simulink model "simulator"  (R2023b)
settings: configuration reference "SharedConfiguration" (kept outside this file)
undefined symbols (not defined in the file or in its folder): DiscIntNeverNeededParam
libraries: simulink x20
(part 1 of 2)
settings Model: DataDictionary=SharedDataDictionary.sldd  PacingRate=0.001000  VariantFading=off  Creator=hubkapatrik  LastModifiedBy=Ja
settings ConfigSetRef: SourceName=SharedConfiguration

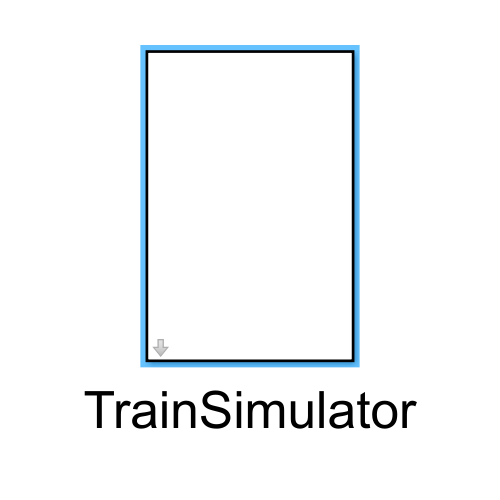
[thumbnail: Simulink's stored preview of the top-level diagram]
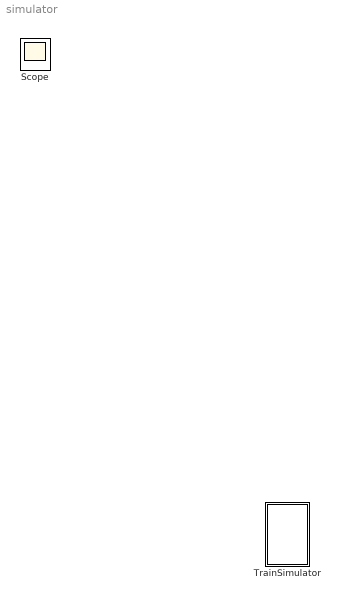
== system simulator ==
  TrainSimulator : Subsystem  mask{VelocityStart=10, MethodOfSpeedChange=constant acceleration, VelocityReq=10, Acceleration=1, PowerMaximum=3, PowerRelative=0.060, TractionForce=300, RoadResistEnable=yes, Gradient=0, CI_AfterReset=1, CI_Overreading=5.0, CI_Underreading=5.0, DrivingDirection=nominal}
      mask prompts: VelocityStart "Initial velocity"; MethodOfSpeedChange "Method of speed change"; VelocityReq "Required velocity"; PowerMaximum "Maximum power [MW]"; PowerRelative "Relative power [-]"; TractionForce "Traction force [kN]"; RoadResistEnable "Road resist enable"; Gradient "Gradient [‰]"; CI_AfterReset "Initial CI [%]"; CI_Overreading "CI overreading [%]"; CI_Underreading "CI underreading [%]"; DrivingDirection "Direction of train"
      mask TypeOptions MethodOfSpeedChange: constant velocity | sudden change of velocity | constant acceleration | break curves (not finished) | traction characteristics (not finished)
      mask TypeOptions RoadResistEnable: yes | no
      mask TypeOptions DrivingDirection: nominal | reverse
      mask DialogControl Container2 Prompt: Constant Acceleration
      mask DialogControl Container3 Prompt: Traction Characteristics
      mask DialogControl Container4 Prompt: Confidence Interval
  Scope : Scope

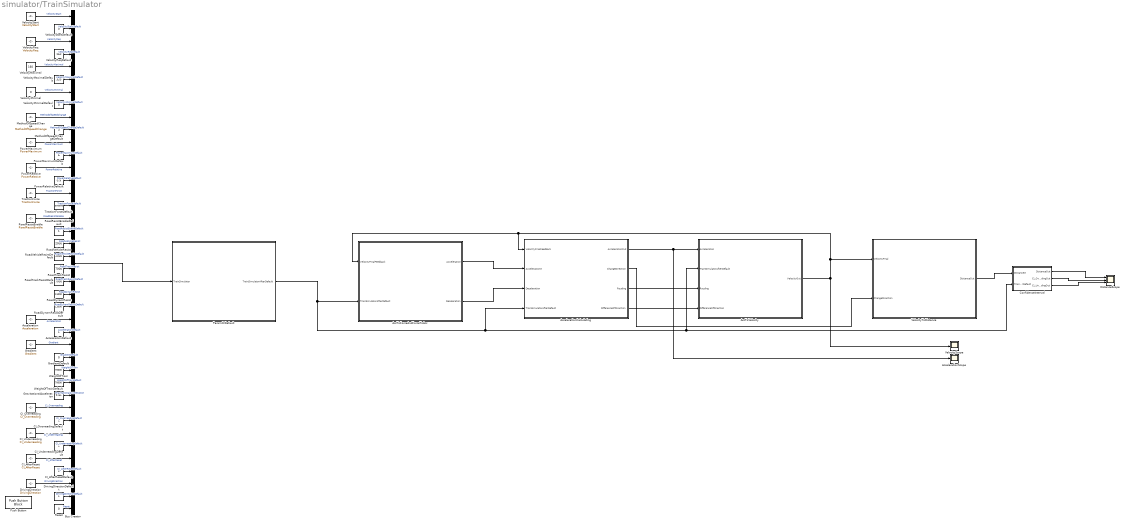
== system simulator/TrainSimulator ==
  AccToForceAndForceToAcc : Subsystem
  AccToVelocity : Subsystem
  Acceleration : Constant  Value=Acceleration  VectorParams1D=off  OutDataTypeStr=double
  AccelerationCalculating : Subsystem
  AccelerationDefault : Constant  VectorParams1D=off  OutDataTypeStr=double
  AccelerationScope : Scope
  Bus Creator : BusCreator  Inputs=VelocityStart,VelocityStartDefault,VelocityReq,VelocityReqDefault,VelocityMaximal,VelocityMaximalDefault,VelocityMinimal,VelocityMinimalDefault,MethodOfSpeedChange,MethodOfSpeedChangeDefault,PowerMaximum,PowerMaximumDefault,PowerRelative,PowerRelativeDefault,TractionForce,TractionForceDefault,RoadResistEnable,RoadResistEnableDefault,RoadVehicleResist,RoadVehicleResistDefault,RoadTrackResist,RoadTrackResistDefault,RoadDynamResist,RoadDynamResistDefault,Acceleration,AccelerationDefault,Gradient,GradientDefault,WeightOfTrain,WeightOfTrainDefault,GravitationalAcceleration,CI_Overreading,CI_OverreadingDefault,CI_Underreading,CI_UnderreadingDefault,CI_AfterReset,CI_AfterResetDefault,DrivingDirection,DrivingDirectionDefault,Reset  OutDataTypeStr=Bus: TrainSimulator  NonVirtualBus=on
  CI_AfterReset : Constant  Value=CI_AfterReset
  CI_AfterResetDefault : Constant  OutDataTypeStr=double
  CI_Overreading : Constant  Value=CI_Overreading
  CI_OverreadingDefault : Constant  OutDataTypeStr=double
  CI_Underreading : Constant  Value=CI_Underreading
  CI_UnderreadingDefault : Constant  OutDataTypeStr=double
  ConfidenceInterval : Subsystem
  DistanceScope : Scope  NumInputPorts=3
  DrivingDirection : Constant  Value=DrivingDirection  OutMin=0  OutMax=2  OutDataTypeStr=uint8
  DrivingDirectionDefault : Constant  OutMin=0  OutMax=2  OutDataTypeStr=uint8
  Gradient : Constant  Value=Gradient  OutDataTypeStr=double
  GradientDefault : Constant  Value=0  OutDataTypeStr=double
  GravitationalAcceleration : Constant  Value=9.81  OutMin=0  OutDataTypeStr=double
  MethodOfSpeedChange : Constant  Value=MethodOfSpeedChange  VectorParams1D=off  OutMin=1  OutMax=5  OutDataTypeStr=double
  MethodOfSpeedChangeDefault : Constant  Value=3  OutMin=1  OutMax=5  OutDataTypeStr=double
  ParamOrDefault : Subsystem
  PowerMaximum : Constant  Value=PowerMaximum
  PowerMaximumDefault : Constant  Value=6
  PowerRelative : Constant  Value=PowerRelative
  PowerRelativeDefault : Constant  Value=0.9
  Push Button : PushButtonBlock  OffValue=0.000000
  Reset : Constant  Value=0  OutMin=0  OutMax=1  OutDataTypeStr=double
  RoadDynamResist : Constant  Value=11000  OutMin=0  OutDataTypeStr=double
  RoadDynamResistDefault : Constant  Value=11000  VectorParams1D=off  OutMin=0  OutDataTypeStr=double
  RoadResistEnable : Constant  Value=RoadResistEnable  OutMin=0  OutMax=2  OutDataTypeStr=double
  RoadResistEnableDefault : Constant  OutMin=0  OutMax=1  OutDataTypeStr=double
  RoadTrackResist : Constant  Value=7000  OutMin=0  OutDataTypeStr=double
  RoadTrackResistDefault : Constant  Value=7000  OutMin=0  OutDataTypeStr=double
  RoadVehicleResist : Constant  Value=2000  OutMin=0  OutDataTypeStr=double
  RoadVehicleResistDefault : Constant  Value=2000  OutMin=0  OutDataTypeStr=double
  TractionForce : Constant  Value=TractionForce
  TractionForceDefault : Constant  Value=300000
  VelocityMaximal : Constant  Value=160  OutMin=0  OutDataTypeStr=double
  VelocityMaximalDefault : Constant  Value=320  OutMin=0  OutDataTypeStr=double
  VelocityMinimal : Constant  Value=0  OutMin=0  OutDataTypeStr=double
  VelocityMinimalDefault : Constant  Value=0  OutMin=0  OutDataTypeStr=double
  VelocityReq : Constant  Value=VelocityReq  OutMin=0  OutDataTypeStr=double
  VelocityReqDefault : Constant  Value=160  OutMin=0  OutDataTypeStr=double
  VelocityScope : Scope
  VelocityStart : Constant  Value=VelocityStart  OutMin=0  OutDataTypeStr=double
  VelocityStartDefault : Constant  Value=0  OutMin=0  OutDataTypeStr=double
  VelocityToDistance : Subsystem
  WeightOfTrain : Constant  Value=70000  OutMin=0  OutDataTypeStr=double
  WeightOfTrainDefault : Constant  Value=70000  OutMin=0  OutDataTypeStr=double
  wires:
  MethodOfSpeedChange/1 -> Bus Creator/9  "MethodOfSpeedChange"
  VelocityReq/1 -> Bus Creator/3  "VelocityReq"
  VelocityToDistance/1(DistanceOut) -> ConfidenceInterval/1(DistanceIn)
  Reset/1 -> Bus Creator/40  "Reset"
  VelocityStartDefault/1 -> Bus Creator/2  "VelocityStartDefault"
  Bus Creator/1 -> ParamOrDefault/1(TrainSimulator)
  DrivingDirectionDefault/1 -> Bus Creator/39  "DrivingDirectionDefault"
  RoadDynamResistDefault/1 -> Bus Creator/24  "RoadDynamResistDefault"
  RoadTrackResist/1 -> Bus Creator/21  "RoadTrackResist"
  RoadResistEnable/1 -> Bus Creator/17  "RoadResistEnable"
  RoadDynamResist/1 -> Bus Creator/23  "RoadDynamResist"
  RoadVehicleResist/1 -> Bus Creator/19  "RoadVehicleResist"
  Acceleration/1 -> Bus Creator/25  "Acceleration"
  ParamOrDefault/1(TrainSimulatorAfterDefault) -> ConfidenceInterval/2(TrainSimulatorAfterDefault), AccToVelocity/2(TrainSimulatorAfterDefault), AccelerationCalculating/4(TrainSimulatorAfterDefault), AccToForceAndForceToAcc/2(TrainSimulatorAfterDefault)
  WeightOfTrain/1 -> Bus Creator/29  "WeightOfTrain"
  RoadResistEnableDefault/1 -> Bus Creator/18  "RoadResistEnableDefault"
  GravitationalAcceleration/1 -> Bus Creator/31  "GravitationalAcceleration"
  MethodOfSpeedChangeDefault/1 -> Bus Creator/10  "MethodOfSpeedChangeDefault"
  GradientDefault/1 -> Bus Creator/28  "GradientDefault"
  AccelerationCalculating/1(AccelerationOut) -> AccelerationScope/1, AccToVelocity/1(Acceleration)
  RoadTrackResistDefault/1 -> Bus Creator/22  "RoadTrackResistDefault"
  VelocityReqDefault/1 -> Bus Creator/4  "VelocityReqDefault"
  WeightOfTrainDefault/1 -> Bus Creator/30  "WeightOfTrainDefault"
  AccToForceAndForceToAcc/1(Acceleration) -> AccelerationCalculating/2(AccelerationIn)
  Gradient/1 -> Bus Creator/27  "Gradient"
  AccelerationCalculating/2(ChangeDirection) -> VelocityToDistance/2(ChangeDirection)
  DrivingDirection/1 -> Bus Creator/38  "DrivingDirection"
  VelocityStart/1 -> Bus Creator/1  "VelocityStart"
  RoadVehicleResistDefault/1 -> Bus Creator/20  "RoadVehicleResistDefault"
  VelocityMinimal/1 -> Bus Creator/7  "VelocityMinimal"
  VelocityMinimalDefault/1 -> Bus Creator/8  "VelocityMinimalDefault"
  AccToForceAndForceToAcc/2(Deceleration) -> AccelerationCalculating/3(Deceleration)
  VelocityMaximal/1 -> Bus Creator/5  "VelocityMaximal"
  VelocityMaximalDefault/1 -> Bus Creator/6  "VelocityMaximalDefault"
  AccToVelocity/1(VelocityOut) -> AccelerationCalculating/1(VelocityFinalFeedback), AccToForceAndForceToAcc/1(VelocityFinalFeedback), VelocityToDistance/1(VelocityFinal), VelocityScope/1
  PowerRelative/1 -> Bus Creator/13  "PowerRelative"
  PowerRelativeDefault/1 -> Bus Creator/14  "PowerRelativeDefault"
  PowerMaximumDefault/1 -> Bus Creator/12  "PowerMaximumDefault"
  PowerMaximum/1 -> Bus Creator/11  "PowerMaximum"
  TractionForceDefault/1 -> Bus Creator/16  "TractionForceDefault"
  TractionForce/1 -> Bus Creator/15  "TractionForce"
  AccelerationCalculating/3(Rouding) -> AccToVelocity/3(Rouding)
  AccelerationCalculating/4(DifferenceOfDirection) -> AccToVelocity/4(DifferenceOfDirection)
  CI_Overreading/1 -> Bus Creator/32  "CI_Overreading"
  CI_Underreading/1 -> Bus Creator/34  "CI_Underreading"
  CI_AfterReset/1 -> Bus Creator/36  "CI_AfterReset"
  ConfidenceInterval/1(DistanceOut) -> DistanceScope/1
  ConfidenceInterval/2(CI_OverreadingOut) -> DistanceScope/2
  ConfidenceInterval/3(CI_UnderreadingOut) -> DistanceScope/3
  AccelerationDefault/1 -> Bus Creator/26  "AccelerationDefault"
  CI_OverreadingDefault/1 -> Bus Creator/33  "CI_OverreadingDefault"
  CI_UnderreadingDefault/1 -> Bus Creator/35  "CI_UnderreadingDefault"
  CI_AfterResetDefault/1 -> Bus Creator/37  "CI_AfterResetDefault"

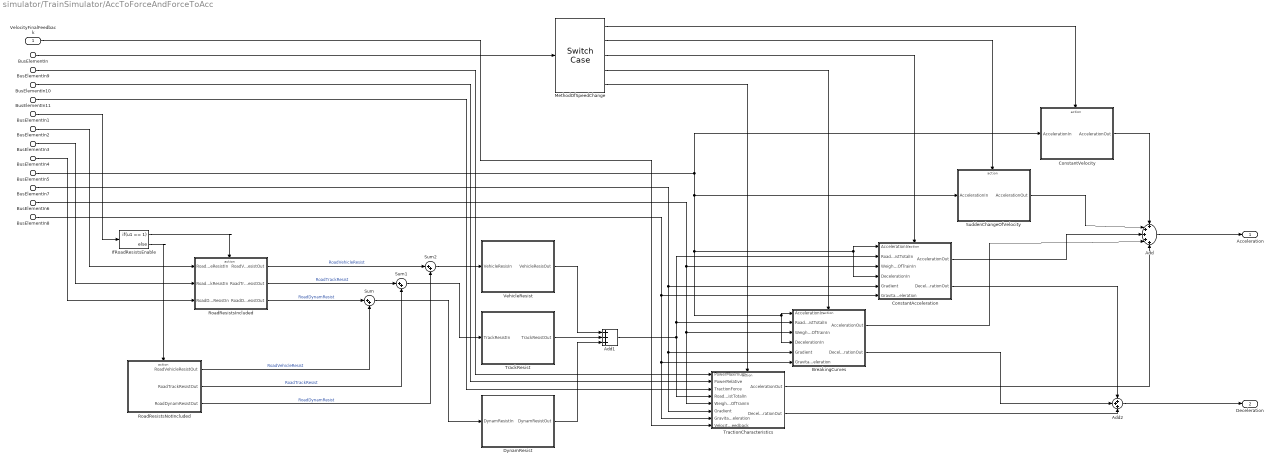
== system simulator/TrainSimulator/AccToForceAndForceToAcc ==
  VelocityFinalFeedback : Inport
  BusElementIn : Inport  Port=2  PortName=TrainSimulatorAfterDefault  Element=MethodOfSpeedChange
  BusElementIn9 : Inport  Port=2  PortName=TrainSimulatorAfterDefault  Element=PowerMaximum
  BusElementIn10 : Inport  Port=2  PortName=TrainSimulatorAfterDefault  Element=PowerRelative
  BusElementIn11 : Inport  Port=2  PortName=TrainSimulatorAfterDefault  Element=TractionForce
  BusElementIn1 : Inport  Port=2  PortName=TrainSimulatorAfterDefault  Element=RoadResistEnable
  BusElementIn2 : Inport  Port=2  PortName=TrainSimulatorAfterDefault  Element=RoadVehicleResist
  BusElementIn3 : Inport  Port=2  PortName=TrainSimulatorAfterDefault  Element=RoadTrackResist
  BusElementIn4 : Inport  Port=2  PortName=TrainSimulatorAfterDefault  Element=RoadDynamResist
  BusElementIn5 : Inport  Port=2  PortName=TrainSimulatorAfterDefault  Element=Acceleration
  BusElementIn7 : Inport  Port=2  PortName=TrainSimulatorAfterDefault  Element=Gradient
  BusElementIn6 : Inport  Port=2  PortName=TrainSimulatorAfterDefault  Element=WeightOfTrain
  BusElementIn8 : Inport  Port=2  PortName=TrainSimulatorAfterDefault  Element=GravitationalAcceleration
  Add : Sum  Inputs=+++++  OutDataTypeStr=double  AccumDataTypeStr=double
  Add1 : Sum  Inputs=+++  OutMin=0  OutDataTypeStr=double  AccumDataTypeStr=double
  Add2 : Sum  Inputs=+++  OutDataTypeStr=double  AccumDataTypeStr=double
  BreakingCurves : Subsystem
  ConstantAcceleration : Subsystem
  ConstantVelocity : Subsystem
  DynamResist : Subsystem
  IfRoadResistsEnable : If  IfExpression=u1 == 1
  MethodOfSpeedChange : SwitchCase  CaseConditions={1,2,3,4,5}  ShowDefaultCase=off
  RoadResistsIncluded : Subsystem
  RoadResistsNotIncluded : Subsystem
  SuddenChangeOfVelocity : Subsystem
  Sum : Sum  Inputs=|++  OutMin=0  AccumDataTypeStr=double
  Sum1 : Sum  Inputs=|++  OutMin=0  AccumDataTypeStr=double
  Sum2 : Sum  Inputs=|++  OutMin=0  AccumDataTypeStr=double
  TrackResist : Subsystem
  TractionCharacteristics : Subsystem
  VehicleResist : Subsystem
  Acceleration : Outport  OutDataTypeStr=double
  Deceleration : Outport  Port=2  OutDataTypeStr=double
  wires:
  BusElementIn/1 -> MethodOfSpeedChange/1
  MethodOfSpeedChange/5 -> TractionCharacteristics/Action
  MethodOfSpeedChange/4 -> BreakingCurves/Action
  MethodOfSpeedChange/3 -> ConstantAcceleration/Action
  MethodOfSpeedChange/2 -> SuddenChangeOfVelocity/Action
  MethodOfSpeedChange/1 -> ConstantVelocity/Action
  BusElementIn5/1 -> BreakingCurves/4(DecelerationIn), BreakingCurves/1(AccelerationIn), ConstantAcceleration/4(DecelerationIn), ConstantAcceleration/1(AccelerationIn), SuddenChangeOfVelocity/1(AccelerationIn), ConstantVelocity/1(AccelerationIn)
  ConstantVelocity/1(AccelerationOut) -> Add/1
  ConstantAcceleration/1(AccelerationOut) -> Add/3
  BreakingCurves/1(AccelerationOut) -> Add/4
  TractionCharacteristics/1(AccelerationOut) -> Add/5
  IfRoadResistsEnable/1 -> RoadResistsIncluded/Action
  IfRoadResistsEnable/2 -> RoadResistsNotIncluded/Action
  RoadResistsNotIncluded/1(RoadVehicleResistOut) -> Sum/2  "RoadVehicleResist"
  RoadResistsNotIncluded/2(RoadTrackResistOut) -> Sum1/2  "RoadTrackResist"
  RoadResistsNotIncluded/3(RoadDynamResistOut) -> Sum2/2  "RoadDynamResist"
  RoadResistsIncluded/1(RoadVehicleResistOut) -> Sum2/1  "RoadVehicleResist"
  RoadResistsIncluded/2(RoadTrackResistOut) -> Sum1/1  "RoadTrackResist"
  RoadResistsIncluded/3(RoadDynamResistOut) -> Sum/1  "RoadDynamResist"
  SuddenChangeOfVelocity/1(AccelerationOut) -> Add/2
  VehicleResist/1(VehicleResisOut) -> Add1/1
  TrackResist/1(TrackResistOut) -> Add1/2
  DynamResist/1(DynamResistOut) -> Add1/3
  Add1/1 -> BreakingCurves/2(RoadResistTotalIn), ConstantAcceleration/2(RoadResistTotalIn), TractionCharacteristics/4(RoadResistTotalIn)
  BusElementIn1/1 -> IfRoadResistsEnable/1
  BusElementIn2/1 -> RoadResistsIncluded/1(RoadVehicleResistIn)
  BusElementIn3/1 -> RoadResistsIncluded/2(RoadTrackResistIn)
  BusElementIn4/1 -> RoadResistsIncluded/3(RoadDynamResistIn)
  BusElementIn6/1 -> ConstantAcceleration/3(WeightOfTrainIn), BreakingCurves/3(WeightOfTrainIn), TractionCharacteristics/5(WeightOfTrainIn)
  ConstantAcceleration/2(DecelerationOut) -> Add2/1
  BreakingCurves/2(DecelerationOut) -> Add2/2
  TractionCharacteristics/2(DecelerationOut) -> Add2/3
  Sum/1 -> DynamResist/1(DynamResistIn)
  Sum1/1 -> TrackResist/1(TrackResistIn)
  Sum2/1 -> VehicleResist/1(VehicleResisIn)
  BusElementIn7/1 -> ConstantAcceleration/5(Gradient), BreakingCurves/5(Gradient), TractionCharacteristics/6(Gradient)
  BusElementIn8/1 -> ConstantAcceleration/6(GravitationalAcceleration), BreakingCurves/6(GravitationalAcceleration), TractionCharacteristics/7(GravitationalAcceleration)
  BusElementIn11/1 -> TractionCharacteristics/3(TractionForce)
  BusElementIn10/1 -> TractionCharacteristics/2(PowerRelative)
  BusElementIn9/1 -> TractionCharacteristics/1(PowerMaximum)
  VelocityFinalFeedback/1 -> TractionCharacteristics/8(VelocityFinalFeedback)
  Add/1 -> Acceleration/1
  Add2/1 -> Deceleration/1

== system simulator/TrainSimulator/AccToVelocity ==
  Acceleration : Inport  OutDataTypeStr=double
  BusElementIn : Inport  Port=2  PortName=TrainSimulatorAfterDefault  Element=VelocityStart
  BusElementIn1 : Inport  Port=2  PortName=TrainSimulatorAfterDefault  Element=VelocityReq
  BusElementIn3 : Inport  Port=2  PortName=TrainSimulatorAfterDefault  Element=VelocityMaximal
  BusElementIn2 : Inport  Port=2  PortName=TrainSimulatorAfterDefault  Element=VelocityMinimal
  Rouding : Inport  Port=3
  DifferenceOfDirection : Inport  Port=4  OutDataTypeStr=boolean
  AND : Logic  AllPortsSameDT=off  OutDataTypeStr=boolean
  Delay : Delay  DelayLength=1  InitialConditionSource=Input port  InitialCondition=20
      settings: InputPortMap=u0,p4
  DynamicChangeLimitMaxMinVelocity : Subsystem
  Switch : Switch  Criteria=u2 > Threshold  SaturateOnIntegerOverflow=off  InputSameDT=off
  VelocityOut : Outport  OutDataTypeStr=double
  wires:
  BusElementIn/1 -> Delay/2, DynamicChangeLimitMaxMinVelocity/3(VelocityStart)
  BusElementIn2/1 -> DynamicChangeLimitMaxMinVelocity/4(VelocityMinimal)
  Acceleration/1 -> DynamicChangeLimitMaxMinVelocity/1(Acceleration)
  BusElementIn3/1 -> DynamicChangeLimitMaxMinVelocity/2(VelocityMaxial)
  BusElementIn1/1 -> Switch/1
  Delay/1 -> VelocityOut/1
  DynamicChangeLimitMaxMinVelocity/1(VelocityOut) -> Switch/3
  AND/1 -> Switch/2
  DifferenceOfDirection/1 -> AND/1
  Switch/1 -> Delay/1
  Rouding/1 -> AND/2

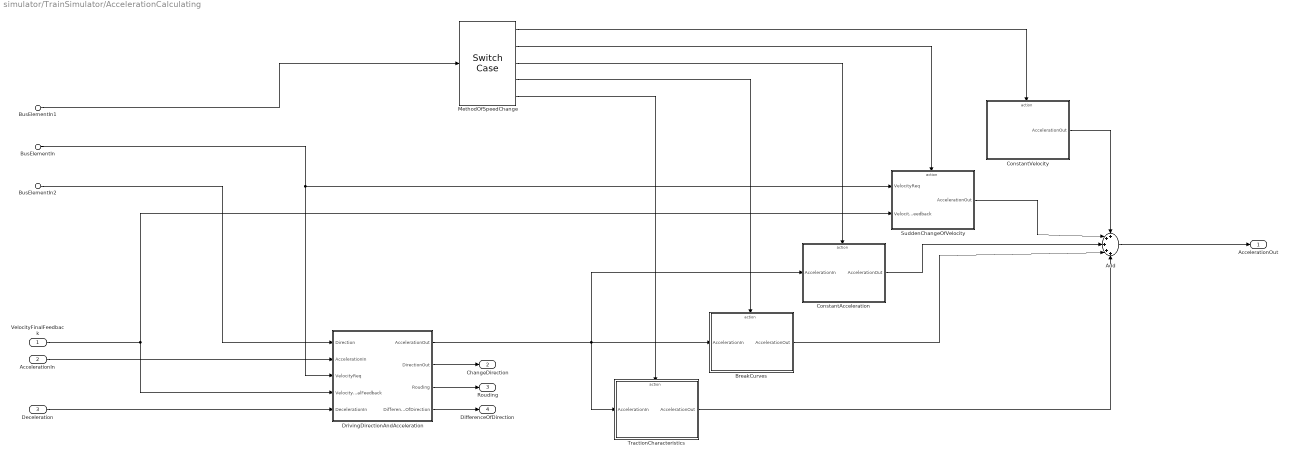
== system simulator/TrainSimulator/AccelerationCalculating ==
  VelocityFinalFeedback : Inport  OutDataTypeStr=double
  AccelerationIn : Inport  Port=2  OutDataTypeStr=double
  Deceleration : Inport  Port=3  OutDataTypeStr=double
  BusElementIn : Inport  Port=4  PortName=TrainSimulatorAfterDefault  Element=VelocityReq
  BusElementIn1 : Inport  Port=4  PortName=TrainSimulatorAfterDefault  Element=MethodOfSpeedChange
  BusElementIn2 : Inport  Port=4  PortName=TrainSimulatorAfterDefault  Element=DrivingDirection
  Add : Sum  Inputs=+++++  OutDataTypeStr=double  AccumDataTypeStr=double
  BreakCurves : Subsystem
  ConstantAcceleration : Subsystem
  ConstantVelocity : Subsystem
  DrivingDirectionAndAcceleration : Subsystem
  MethodOfSpeedChange : SwitchCase  CaseConditions={1,2,3,4,5}  ShowDefaultCase=off
  SuddenChangeOfVelocity : Subsystem
  TractionCharacteristics : Subsystem
  AccelerationOut : Outport  OutDataTypeStr=double
  ChangeDirection : Outport  Port=2  OutDataTypeStr=uint8
  Rouding : Outport  Port=3  OutDataTypeStr=double
  DifferenceOfDirection : Outport  Port=4  OutDataTypeStr=boolean
  wires:
  MethodOfSpeedChange/5 -> TractionCharacteristics/Action
  MethodOfSpeedChange/4 -> BreakCurves/Action
  MethodOfSpeedChange/3 -> ConstantAcceleration/Action
  MethodOfSpeedChange/1 -> ConstantVelocity/Action
  ConstantVelocity/1(AccelerationOut) -> Add/1
  SuddenChangeOfVelocity/1(AccelerationOut) -> Add/2
  ConstantAcceleration/1(AccelerationOut) -> Add/3
  TractionCharacteristics/1(AccelerationOut) -> Add/5
  MethodOfSpeedChange/2 -> SuddenChangeOfVelocity/Action
  BreakCurves/1(AccelerationOut) -> Add/4
  BusElementIn1/1 -> MethodOfSpeedChange/1
  BusElementIn2/1 -> DrivingDirectionAndAcceleration/1(Direction)
  BusElementIn/1 -> DrivingDirectionAndAcceleration/3(VelocityReq), SuddenChangeOfVelocity/1(VelocityReq)
  DrivingDirectionAndAcceleration/1(AccelerationOut) -> ConstantAcceleration/1(AccelerationIn), TractionCharacteristics/1(AccelerationIn), BreakCurves/1(AccelerationIn)
  AccelerationIn/1 -> DrivingDirectionAndAcceleration/2(AccelerationIn)
  VelocityFinalFeedback/1 -> DrivingDirectionAndAcceleration/4(VelocityFinalFeedback), SuddenChangeOfVelocity/2(VelocityFinalFeedback)
  Add/1 -> AccelerationOut/1
  DrivingDirectionAndAcceleration/2(DirectionOut) -> ChangeDirection/1
  Deceleration/1 -> DrivingDirectionAndAcceleration/5(DecelerationIn)
  DrivingDirectionAndAcceleration/3(Rouding) -> Rouding/1
  DrivingDirectionAndAcceleration/4(DifferenceOfDirection) -> DifferenceOfDirection/1

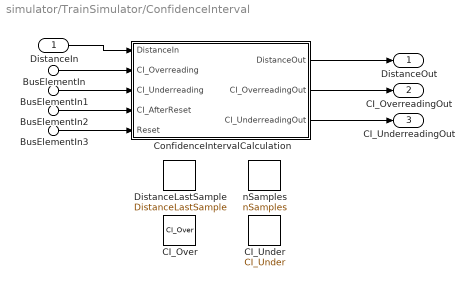
== system simulator/TrainSimulator/ConfidenceInterval ==
  DistanceIn : Inport  OutDataTypeStr=double
  BusElementIn : Inport  Port=2  PortName=TrainSimulatorAfterDefault  Element=CI_Overreading
  BusElementIn1 : Inport  Port=2  PortName=TrainSimulatorAfterDefault  Element=CI_Underreading
  BusElementIn2 : Inport  Port=2  PortName=TrainSimulatorAfterDefault  Element=CI_AfterReset
  BusElementIn3 : Inport  Port=2  PortName=TrainSimulatorAfterDefault  Element=Reset
  CI_Over : DataStoreMemory  DataStoreName=CI_Over  WriteAfterWriteMsg=warning  ShowAdditionalParam=off  OutDataTypeStr=double
  CI_Under : DataStoreMemory  DataStoreName=CI_Under  WriteAfterWriteMsg=warning  ShowAdditionalParam=off  OutDataTypeStr=double
  ConfidenceIntervalCalculation : MATLAB Function  TreatAsAtomicUnit=on
  DistanceLastSample : DataStoreMemory  DataStoreName=DistanceLastSample  WriteAfterWriteMsg=warning  ShowAdditionalParam=off  OutDataTypeStr=double
  nSamples : DataStoreMemory  DataStoreName=nSamples  WriteAfterWriteMsg=warning  ShowAdditionalParam=off  OutDataTypeStr=double
  DistanceOut : Outport
  CI_OverreadingOut : Outport  Port=2
  CI_UnderreadingOut : Outport  Port=3
  wires:
  BusElementIn3/1 -> ConfidenceIntervalCalculation/5(Reset)
  BusElementIn2/1 -> ConfidenceIntervalCalculation/4(CI_AfterReset)
  BusElementIn1/1 -> ConfidenceIntervalCalculation/3(CI_Underreading)
  BusElementIn/1 -> ConfidenceIntervalCalculation/2(CI_Overreading)
  DistanceIn/1 -> ConfidenceIntervalCalculation/1(DistanceIn)
  ConfidenceIntervalCalculation/2(CI_OverreadingOut) -> CI_OverreadingOut/1
  ConfidenceIntervalCalculation/1(DistanceOut) -> DistanceOut/1
  ConfidenceIntervalCalculation/3(CI_UnderreadingOut) -> CI_UnderreadingOut/1

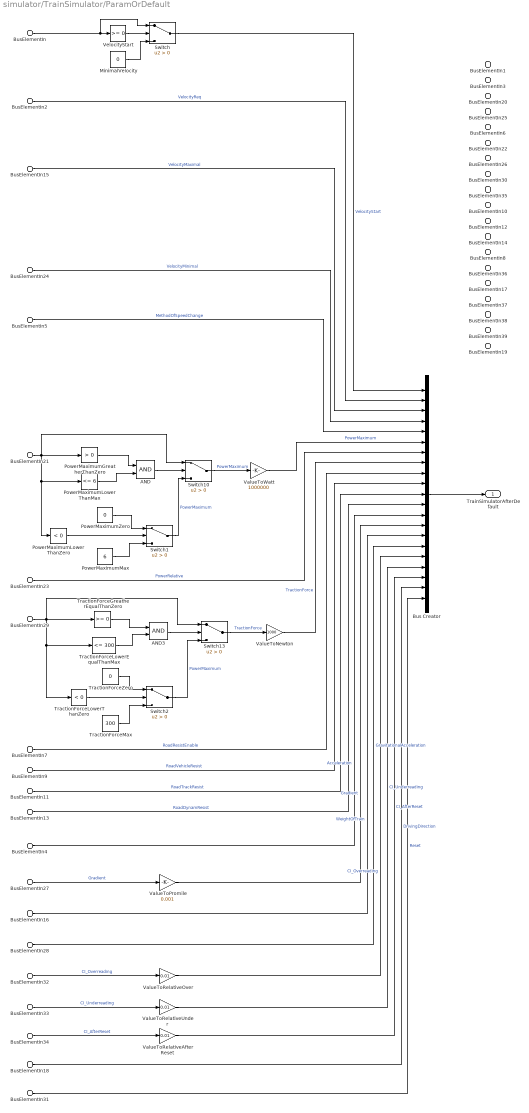
== system simulator/TrainSimulator/ParamOrDefault ==
  BusElementIn : Inport  PortName=TrainSimulator  Element=VelocityStart
  BusElementIn1 : Inport  PortName=TrainSimulator  Element=VelocityStartDefault
  BusElementIn2 : Inport  PortName=TrainSimulator  Element=VelocityReq
  BusElementIn3 : Inport  PortName=TrainSimulator  Element=VelocityReqDefault
  BusElementIn15 : Inport  PortName=TrainSimulator  Element=VelocityMaximal
  BusElementIn20 : Inport  PortName=TrainSimulator  Element=VelocityMaximalDefault
  BusElementIn24 : Inport  PortName=TrainSimulator  Element=VelocityMinimal
  BusElementIn25 : Inport  PortName=TrainSimulator  Element=VelocityMinimalDefault
  BusElementIn5 : Inport  PortName=TrainSimulator  Element=MethodOfSpeedChange
  BusElementIn6 : Inport  PortName=TrainSimulator  Element=MethodOfSpeedChangeDefault
  BusElementIn21 : Inport  PortName=TrainSimulator  Element=PowerMaximum
  BusElementIn22 : Inport  PortName=TrainSimulator  Element=PowerMaximumDefault
  BusElementIn23 : Inport  PortName=TrainSimulator  Element=PowerRelative
  BusElementIn26 : Inport  PortName=TrainSimulator  Element=PowerRelativeDefault
  BusElementIn29 : Inport  PortName=TrainSimulator  Element=TractionForce
  BusElementIn30 : Inport  PortName=TrainSimulator  Element=TractionForceDefault
  BusElementIn7 : Inport  PortName=TrainSimulator  Element=RoadResistEnable
  BusElementIn35 : Inport  PortName=TrainSimulator  Element=RoadResistEnableDefault
  BusElementIn9 : Inport  PortName=TrainSimulator  Element=RoadVehicleResist
  BusElementIn10 : Inport  PortName=TrainSimulator  Element=RoadVehicleResistDefault
  BusElementIn11 : Inport  PortName=TrainSimulator  Element=RoadTrackResist
  BusElementIn12 : Inport  PortName=TrainSimulator  Element=RoadTrackResistDefault
  BusElementIn13 : Inport  PortName=TrainSimulator  Element=RoadDynamResist
  BusElementIn14 : Inport  PortName=TrainSimulator  Element=RoadDynamResistDefault
  BusElementIn4 : Inport  PortName=TrainSimulator  Element=Acceleration
  BusElementIn8 : Inport  PortName=TrainSimulator  Element=AccelerationDefault
  BusElementIn27 : Inport  PortName=TrainSimulator  Element=Gradient
  BusElementIn36 : Inport  PortName=TrainSimulator  Element=GradientDefault
  BusElementIn16 : Inport  PortName=TrainSimulator  Element=WeightOfTrain
  BusElementIn17 : Inport  PortName=TrainSimulator  Element=WeightOfTrainDefault
  BusElementIn28 : Inport  PortName=TrainSimulator  Element=GravitationalAcceleration
  BusElementIn32 : Inport  PortName=TrainSimulator  Element=CI_Overreading
  BusElementIn37 : Inport  PortName=TrainSimulator  Element=CI_OverreadingDefault
  BusElementIn33 : Inport  PortName=TrainSimulator  Element=CI_Underreading
  BusElementIn38 : Inport  PortName=TrainSimulator  Element=CI_UnderreadingDefault
  BusElementIn34 : Inport  PortName=TrainSimulator  Element=CI_AfterReset
  BusElementIn39 : Inport  PortName=TrainSimulator  Element=CI_AfterResetDefault
  BusElementIn18 : Inport  PortName=TrainSimulator  Element=DrivingDirection
  BusElementIn19 : Inport  PortName=TrainSimulator  Element=DrivingDirectionDefault
  BusElementIn31 : Inport  PortName=TrainSimulator  Element=Reset
  AND : Logic  AllPortsSameDT=off  OutDataTypeStr=boolean
  AND3 : Logic  AllPortsSameDT=off  OutDataTypeStr=boolean
  Bus Creator : BusCreator  Inputs=21  OutDataTypeStr=Bus: TrainSimulatorAfterDefault  NonVirtualBus=on
  MinimalVelocity : Constant  Value=0  OutDataTypeStr=double
  PowerMaximumGreatherThanZero : simulink/Logic and Bit Operations/Compare To Constant  relop=>  const=0  OutDataTypeStr=boolean
  PowerMaximumLowerThanMax : simulink/Logic and Bit Operations/Compare To Constant  relop=<=  const=6  OutDataTypeStr=boolean
  PowerMaximumLowerThanZero : simulink/Logic and Bit Operations/Compare To Constant  relop=<  const=0  OutDataTypeStr=boolean
  PowerMaximumMax : Constant  Value=6  OutDataTypeStr=double
  PowerMaximumZero : Constant  Value=0  OutDataTypeStr=double
  Switch{,1..2,10} (4 alike) : Switch  Criteria=u2 > Threshold  OutMin=0  OutDataTypeStr=double  SaturateOnIntegerOverflow=off  InputSameDT=off
  Switch13 : Switch  Criteria=u2 > Threshold  OutMin=0  OutMax=1  OutDataTypeStr=double  SaturateOnIntegerOverflow=off  InputSameDT=off
  TractionForceGreatherEqualThanZero : simulink/Logic and Bit Operations/Compare To Constant  relop=>=  const=0  OutDataTypeStr=boolean
  TractionForceLowerEqualThanMax : simulink/Logic and Bit Operations/Compare To Constant  relop=<=  const=300  OutDataTypeStr=boolean
  TractionForceLowerThanZero : simulink/Logic and Bit Operations/Compare To Constant  relop=<  const=0  OutDataTypeStr=boolean
  TractionForceMax : Constant  Value=300  OutDataTypeStr=double
  TractionForceZero : Constant  Value=0  OutDataTypeStr=double
  ValueToNewton : Gain  Gain=1000  ParamDataTypeStr=double  OutDataTypeStr=double
  ValueToPromile : Gain  Gain=0.001  ParamDataTypeStr=double  OutDataTypeStr=double
  ValueToRelativeAfterReset : Gain  Gain=0.01  ParamDataTypeStr=double  OutDataTypeStr=double
  ValueToRelativeOver : Gain  Gain=0.01  ParamDataTypeStr=double  OutDataTypeStr=double
  ValueToRelativeUnder : Gain  Gain=0.01  ParamDataTypeStr=double  OutDataTypeStr=double
  ValueToWatt : Gain  Gain=1000000  ParamDataTypeStr=double  OutDataTypeStr=double
  VelocityStart : simulink/Logic and Bit Operations/Compare To Constant  relop=>=  const=0  OutDataTypeStr=boolean
  TrainSimulatorAfterDefault : Outport  OutDataTypeStr=Bus: TrainSimulatorAfterDefault
  wires:
  VelocityStart/1 -> Switch/2
  Switch/1 -> Bus Creator/1  "VelocityStart"
  BusElementIn2/1 -> Bus Creator/2  "VelocityReq"
  BusElementIn7/1 -> Bus Creator/9  "RoadResistEnable"
  BusElementIn9/1 -> Bus Creator/10  "RoadVehicleResist"
  BusElementIn11/1 -> Bus Creator/11  "RoadTrackResist"
  BusElementIn13/1 -> Bus Creator/12  "RoadDynamResist"
  BusElementIn4/1 -> Bus Creator/13  "Acceleration"
  BusElementIn16/1 -> Bus Creator/15  "WeightOfTrain"
  BusElementIn18/1 -> Bus Creator/20  "DrivingDirection"
  Bus Creator/1 -> TrainSimulatorAfterDefault/1
  BusElementIn5/1 -> Bus Creator/5  "MethodOfSpeedChange"
  BusElementIn/1 -> Switch/1, VelocityStart/1
  BusElementIn24/1 -> Bus Creator/4  "VelocityMinimal"
  BusElementIn15/1 -> Bus Creator/3  "VelocityMaximal"
  BusElementIn21/1 -> PowerMaximumGreatherThanZero/1, Switch10/1, PowerMaximumLowerThanZero/1, PowerMaximumLowerThanMax/1
  ValueToWatt/1 -> Bus Creator/6  "PowerMaximum"
  BusElementIn23/1 -> Bus Creator/7  "PowerRelative"
  BusElementIn28/1 -> Bus Creator/16  "GravitationalAcceleration"
  ValueToPromile/1 -> Bus Creator/14  "Gradient"
  TractionForceGreatherEqualThanZero/1 -> AND3/1
  TractionForceLowerEqualThanMax/1 -> AND3/2
  AND3/1 -> Switch13/2
  ValueToNewton/1 -> Bus Creator/8  "TractionForce"
  BusElementIn31/1 -> Bus Creator/21  "Reset"
  ValueToRelativeOver/1 -> Bus Creator/17  "CI_Overreading"
  ValueToRelativeUnder/1 -> Bus Creator/18  "CI_Underreading"
  ValueToRelativeAfterReset/1 -> Bus Creator/19  "CI_AfterReset"
  Switch10/1 -> ValueToWatt/1  "PowerMaximum"
  Switch13/1 -> ValueToNewton/1  "TractionForce"
  BusElementIn27/1 -> ValueToPromile/1  "Gradient"
  BusElementIn32/1 -> ValueToRelativeOver/1  "CI_Overreading"
  BusElementIn33/1 -> ValueToRelativeUnder/1  "CI_Underreading"
  BusElementIn34/1 -> ValueToRelativeAfterReset/1  "CI_AfterReset"
  MinimalVelocity/1 -> Switch/3
  PowerMaximumGreatherThanZero/1 -> AND/1
  PowerMaximumLowerThanMax/1 -> AND/2
  AND/1 -> Switch10/2
  PowerMaximumLowerThanZero/1 -> Switch1/2
  PowerMaximumZero/1 -> Switch1/1
  PowerMaximumMax/1 -> Switch1/3
  Switch1/1 -> Switch10/3  "PowerMaximum"
  Switch2/1 -> Switch13/3  "PowerMaximum"
  TractionForceZero/1 -> Switch2/1
  BusElementIn29/1 -> TractionForceGreatherEqualThanZero/1, Switch13/1, TractionForceLowerEqualThanMax/1, TractionForceLowerThanZero/1
  TractionForceMax/1 -> Switch2/3
  TractionForceLowerThanZero/1 -> Switch2/2

== system simulator/TrainSimulator/VelocityToDistance ==
  VelocityFinal : Inport  OutDataTypeStr=double
  ChangeDirection : Inport  Port=2  OutDataTypeStr=uint8
  AddOrSubtract : Switch  Criteria=u2 > Threshold  OutDataTypeStr=double  SaturateOnIntegerOverflow=off  InputSameDT=off
  DrivingDirectionNominal : simulink/Logic and Bit Operations/Compare To Constant  relop===  const=2  OutDataTypeStr=boolean
  IfReverseDirectionSubtract : Gain  Gain=-1  OutDataTypeStr=double
  VelocityToDistance : DiscreteIntegrator  IntegratorMethod=Integration: Trapezoidal  gainval=1  SampleTime=-1  OutDataTypeStr=double  ICPrevOutput=DiscIntNeverNeededParam  ICPrevScaledInput=DiscIntNeverNeededParam
  DistanceOut : Outport  OutDataTypeStr=double
  wires:
  VelocityToDistance/1 -> DistanceOut/1
  VelocityFinal/1 -> IfReverseDirectionSubtract/1, AddOrSubtract/3
  IfReverseDirectionSubtract/1 -> AddOrSubtract/1
  AddOrSubtract/1 -> VelocityToDistance/1
  ChangeDirection/1 -> DrivingDirectionNominal/1
  DrivingDirectionNominal/1 -> AddOrSubtract/2

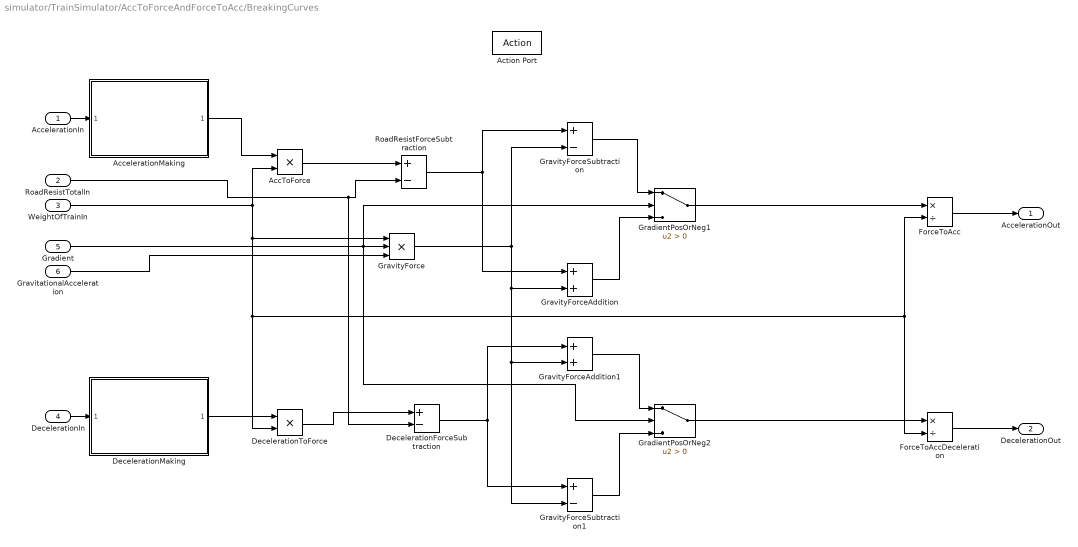
== system simulator/TrainSimulator/AccToForceAndForceToAcc/BreakingCurves ==
  AccelerationIn : Inport  OutDataTypeStr=double
  RoadResistTotalIn : Inport  Port=2  OutDataTypeStr=double
  WeightOfTrainIn : Inport  Port=3  OutDataTypeStr=double
  DecelerationIn : Inport  Port=4  OutDataTypeStr=double
  Gradient : Inport  Port=5
  GravitationalAcceleration : Inport  Port=6
  Action Port : ActionPort  ActionPortLabel=case [ 4 ]:
  AccToForce : Product  OutDataTypeStr=double
  AccelerationMaking : Subsystem  ReferencedSubsystem=AccelerationMaking
  DecelerationForceSubtraction : Sum  Inputs=+-  OutDataTypeStr=double  AccumDataTypeStr=double  RndMeth=Round
  DecelerationMaking : Subsystem  ReferencedSubsystem=DecelerationMaking
  DecelerationToForce : Product  OutDataTypeStr=double
  ForceToAcc : Product  Inputs=*/  OutDataTypeStr=double  RndMeth=Round
  ForceToAccDeceleration : Product  Inputs=*/  OutDataTypeStr=double  RndMeth=Round
  GradientPosOrNeg1 : Switch  Criteria=u2 > Threshold  OutDataTypeStr=double  SaturateOnIntegerOverflow=off  InputSameDT=off
  GradientPosOrNeg2 : Switch  Criteria=u2 > Threshold  OutDataTypeStr=double  SaturateOnIntegerOverflow=off  InputSameDT=off
  GravityForce : Product  Inputs=3  OutDataTypeStr=double
  GravityForceAddition : Sum  OutDataTypeStr=double  AccumDataTypeStr=double  RndMeth=Round
  GravityForceAddition1 : Sum  OutDataTypeStr=double  AccumDataTypeStr=double  RndMeth=Round
  GravityForceSubtraction : Sum  Inputs=+-  OutDataTypeStr=double  AccumDataTypeStr=double  RndMeth=Round
  GravityForceSubtraction1 : Sum  Inputs=+-  OutDataTypeStr=double  AccumDataTypeStr=double  RndMeth=Round
  RoadResistForceSubtraction : Sum  Inputs=+-  OutDataTypeStr=double  AccumDataTypeStr=double  RndMeth=Round
  AccelerationOut : Outport  OutDataTypeStr=double  OutputWhenDisabled=reset  InitialOutput=0
  DecelerationOut : Outport  Port=2  OutDataTypeStr=double  OutputWhenDisabled=reset  InitialOutput=0
  wires:
  DecelerationForceSubtraction/1 -> GravityForceAddition1/1, GravityForceSubtraction1/1
  GravityForceAddition1/1 -> GradientPosOrNeg2/1
  GravityForceSubtraction1/1 -> GradientPosOrNeg2/3
  GradientPosOrNeg2/1 -> ForceToAccDeceleration/1
  GravityForceAddition/1 -> GradientPosOrNeg1/3
  GradientPosOrNeg1/1 -> ForceToAcc/1
  GravityForceSubtraction/1 -> GradientPosOrNeg1/1
  GravityForce/1 -> GravityForceSubtraction/2, GravityForceAddition/2, GravityForceAddition1/2, GravityForceSubtraction1/2
  GravitationalAcceleration/1 -> GravityForce/3
  Gradient/1 -> GradientPosOrNeg1/2, GradientPosOrNeg2/2, GravityForce/2
  RoadResistForceSubtraction/1 -> GravityForceAddition/1, GravityForceSubtraction/1
  AccelerationMaking/1 -> AccToForce/1
  AccelerationIn/1 -> AccelerationMaking/1
  DecelerationMaking/1 -> DecelerationToForce/1
  DecelerationIn/1 -> DecelerationMaking/1
  ForceToAccDeceleration/1 -> DecelerationOut/1
  DecelerationToForce/1 -> DecelerationForceSubtraction/1
  RoadResistTotalIn/1 -> DecelerationForceSubtraction/2, RoadResistForceSubtraction/2
  ForceToAcc/1 -> AccelerationOut/1
  AccToForce/1 -> RoadResistForceSubtraction/1
  WeightOfTrainIn/1 -> AccToForce/2, ForceToAcc/2, ForceToAccDeceleration/2, DecelerationToForce/2, GravityForce/1

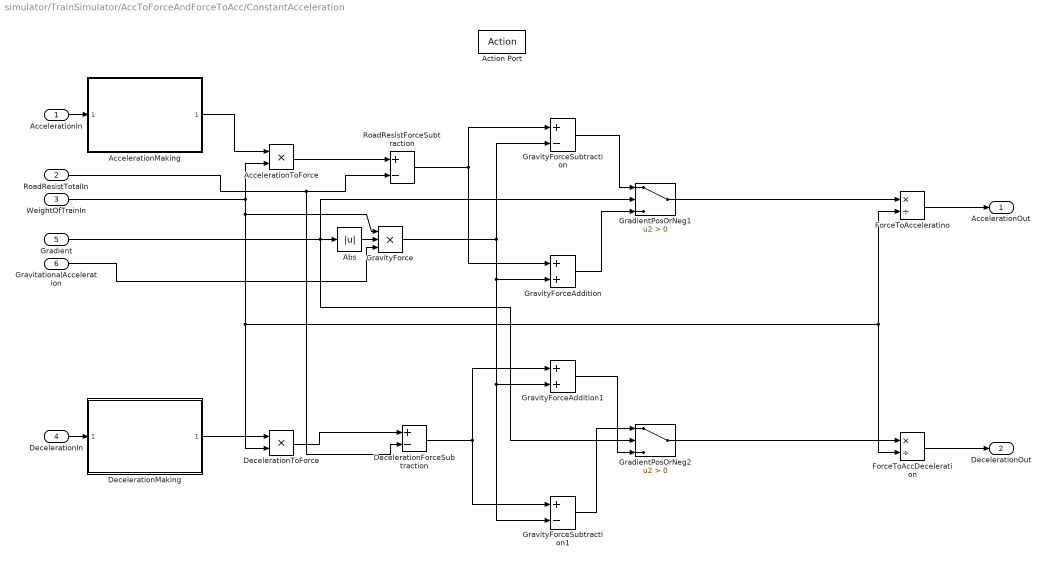
== system simulator/TrainSimulator/AccToForceAndForceToAcc/ConstantAcceleration ==
  AccelerationIn : Inport  OutDataTypeStr=double
  RoadResistTotalIn : Inport  Port=2  OutDataTypeStr=double
  WeightOfTrainIn : Inport  Port=3  OutDataTypeStr=double
  DecelerationIn : Inport  Port=4  OutDataTypeStr=double
  Gradient : Inport  Port=5
  GravitationalAcceleration : Inport  Port=6
  Action Port : ActionPort  ActionPortLabel=case [ 3 ]:
  Abs : Abs  OutDataTypeStr=double  SaturateOnIntegerOverflow=off
  AccelerationMaking : Subsystem  ReferencedSubsystem=AccelerationMaking
  AccelerationToForce : Product  OutDataTypeStr=double
  DecelerationForceSubtraction : Sum  Inputs=+-  OutDataTypeStr=double  AccumDataTypeStr=double  RndMeth=Round
  DecelerationMaking : Subsystem  ReferencedSubsystem=DecelerationMaking
  DecelerationToForce : Product  OutDataTypeStr=double
  ForceToAccDeceleration : Product  Inputs=*/  OutDataTypeStr=double  RndMeth=Round
  ForceToAcceleratino : Product  Inputs=*/  OutDataTypeStr=double  RndMeth=Round
  GradientPosOrNeg1 : Switch  Criteria=u2 > Threshold  OutDataTypeStr=double  SaturateOnIntegerOverflow=off  InputSameDT=off
  GradientPosOrNeg2 : Switch  Criteria=u2 > Threshold  OutDataTypeStr=double  SaturateOnIntegerOverflow=off  InputSameDT=off
  GravityForce : Product  Inputs=3  OutDataTypeStr=double
  GravityForceAddition : Sum  OutDataTypeStr=double  AccumDataTypeStr=double  RndMeth=Round
  GravityForceAddition1 : Sum  OutDataTypeStr=double  AccumDataTypeStr=double  RndMeth=Round
  GravityForceSubtraction : Sum  Inputs=+-  OutDataTypeStr=double  AccumDataTypeStr=double  RndMeth=Round
  GravityForceSubtraction1 : Sum  Inputs=+-  OutDataTypeStr=double  AccumDataTypeStr=double  RndMeth=Round
  RoadResistForceSubtraction : Sum  Inputs=+-  OutDataTypeStr=double  AccumDataTypeStr=double  RndMeth=Round
  AccelerationOut : Outport  OutDataTypeStr=double  OutputWhenDisabled=reset  InitialOutput=0
  DecelerationOut : Outport  Port=2  OutDataTypeStr=double  OutputWhenDisabled=reset  InitialOutput=0
  wires:
  WeightOfTrainIn/1 -> DecelerationToForce/2, ForceToAccDeceleration/2, ForceToAcceleratino/2, GravityForce/1, AccelerationToForce/2
  AccelerationToForce/1 -> RoadResistForceSubtraction/1
  ForceToAcceleratino/1 -> AccelerationOut/1
  RoadResistTotalIn/1 -> RoadResistForceSubtraction/2, DecelerationForceSubtraction/2
  DecelerationToForce/1 -> DecelerationForceSubtraction/1
  ForceToAccDeceleration/1 -> DecelerationOut/1
  DecelerationIn/1 -> DecelerationMaking/1
  DecelerationMaking/1 -> DecelerationToForce/1
  AccelerationIn/1 -> AccelerationMaking/1
  AccelerationMaking/1 -> AccelerationToForce/1
  RoadResistForceSubtraction/1 -> GravityForceSubtraction/1, GravityForceAddition/1
  GravitationalAcceleration/1 -> GravityForce/3
  GravityForce/1 -> GravityForceSubtraction1/2, GravityForceAddition1/2, GravityForceAddition/2, GravityForceSubtraction/2
  GravityForceSubtraction/1 -> GradientPosOrNeg1/1
  GradientPosOrNeg1/1 -> ForceToAcceleratino/1
  GravityForceAddition/1 -> GradientPosOrNeg1/3
  GradientPosOrNeg2/1 -> ForceToAccDeceleration/1
  GravityForceSubtraction1/1 -> GradientPosOrNeg2/1
  GravityForceAddition1/1 -> GradientPosOrNeg2/3
  DecelerationForceSubtraction/1 -> GravityForceSubtraction1/1, GravityForceAddition1/1
  Gradient/1 -> Abs/1, GradientPosOrNeg2/2, GradientPosOrNeg1/2
  Abs/1 -> GravityForce/2

== system simulator/TrainSimulator/AccToForceAndForceToAcc/ConstantVelocity ==
  AccelerationIn : Inport  OutDataTypeStr=double
  Action Port : ActionPort  ActionPortLabel=case [ 1 ]:
  AccelerationOut : Outport  OutDataTypeStr=double  OutputWhenDisabled=reset  InitialOutput=0
  wires:
  AccelerationIn/1 -> AccelerationOut/1

== system simulator/TrainSimulator/AccToForceAndForceToAcc/DynamResist ==
  DynamResistIn : Inport  OutMin=0  OutDataTypeStr=double
  DynamResistOut : Outport  OutMin=0  OutDataTypeStr=double
  wires:
  DynamResistIn/1 -> DynamResistOut/1

== system simulator/TrainSimulator/AccToForceAndForceToAcc/RoadResistsIncluded ==
  RoadVehicleResistIn : Inport  OutMin=0  OutDataTypeStr=double
  RoadTrackResistIn : Inport  Port=2  OutMin=0  OutDataTypeStr=double
  RoadDynamResistIn : Inport  Port=3  OutMin=0  OutDataTypeStr=double
  Action Port : ActionPort  ActionPortLabel=if(u1 == 1)
  RoadVehicleResistOut : Outport  OutMin=0  OutDataTypeStr=double  OutputWhenDisabled=reset  InitialOutput=0
  RoadTrackResistOut : Outport  Port=2  OutMin=0  OutDataTypeStr=double  OutputWhenDisabled=reset  InitialOutput=0
  RoadDynamResistOut : Outport  Port=3  OutMin=0  OutDataTypeStr=double  OutputWhenDisabled=reset  InitialOutput=0
  wires:
  RoadVehicleResistIn/1 -> RoadVehicleResistOut/1
  RoadTrackResistIn/1 -> RoadTrackResistOut/1
  RoadDynamResistIn/1 -> RoadDynamResistOut/1

== system simulator/TrainSimulator/AccToForceAndForceToAcc/RoadResistsNotIncluded ==
  Action Port : ActionPort  ActionPortLabel=else
  RoadDynamResistZero : Constant  Value=0  OutMin=0  OutMax=0  OutDataTypeStr=uint8
  RoadTrackResistZero : Constant  Value=0  OutMin=0  OutMax=0  OutDataTypeStr=uint8
  RoadVehicleResistZero : Constant  Value=0  OutMin=0  OutMax=0  OutDataTypeStr=uint8
  RoadVehicleResistOut : Outport  OutMin=0  OutMax=0  OutDataTypeStr=uint8  OutputWhenDisabled=reset  InitialOutput=0
  RoadTrackResistOut : Outport  Port=2  OutMin=0  OutMax=0  OutDataTypeStr=uint8  OutputWhenDisabled=reset  InitialOutput=0
  RoadDynamResistOut : Outport  Port=3  OutMin=0  OutMax=0  OutDataTypeStr=uint8  OutputWhenDisabled=reset  InitialOutput=0
  wires:
  RoadDynamResistZero/1 -> RoadDynamResistOut/1
  RoadVehicleResistZero/1 -> RoadVehicleResistOut/1
  RoadTrackResistZero/1 -> RoadTrackResistOut/1

== system simulator/TrainSimulator/AccToForceAndForceToAcc/SuddenChangeOfVelocity ==
  AccelerationIn : Inport  OutDataTypeStr=double
  Action Port : ActionPort  ActionPortLabel=case [ 2 ]:
  AccelerationOut : Outport  OutDataTypeStr=double  OutputWhenDisabled=reset  InitialOutput=0
  wires:
  AccelerationIn/1 -> AccelerationOut/1

== system simulator/TrainSimulator/AccToForceAndForceToAcc/TrackResist ==
  TrackResistIn : Inport  OutMin=0  OutDataTypeStr=double
  TrackResistOut : Outport  OutMin=0  OutDataTypeStr=double
  wires:
  TrackResistIn/1 -> TrackResistOut/1

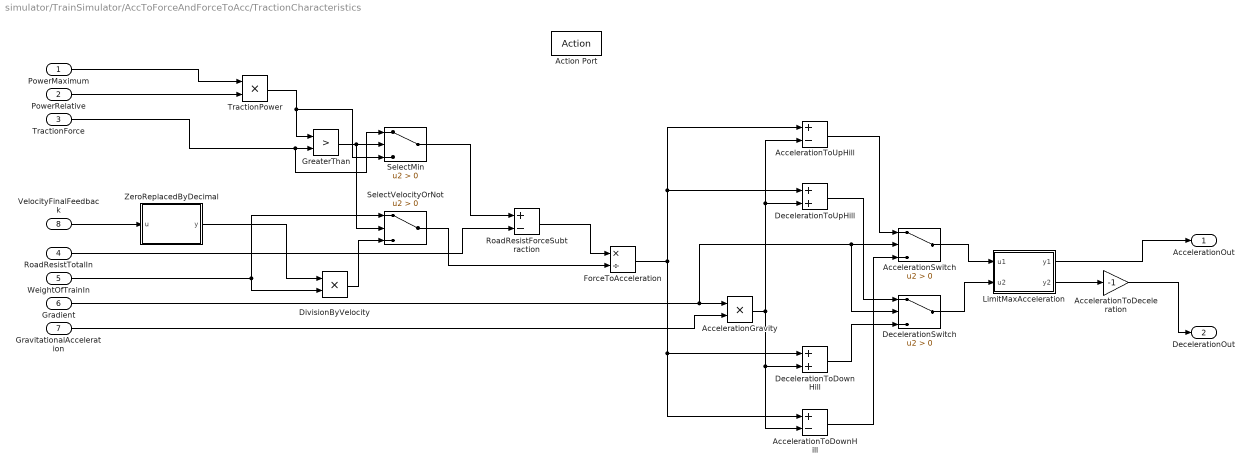
== system simulator/TrainSimulator/AccToForceAndForceToAcc/TractionCharacteristics ==
  PowerMaximum : Inport  OutDataTypeStr=double
  PowerRelative : Inport  Port=2  OutDataTypeStr=double
  TractionForce : Inport  Port=3  OutDataTypeStr=double
  RoadResistTotalIn : Inport  Port=4  OutDataTypeStr=double
  WeightOfTrainIn : Inport  Port=5  OutDataTypeStr=double
  Gradient : Inport  Port=6
  GravitationalAcceleration : Inport  Port=7
  VelocityFinalFeedback : Inport  Port=8
  Action Port : ActionPort  ActionPortLabel=case [ 5 ]:
  AccelerationGravity : Product  OutDataTypeStr=double
  AccelerationSwitch : Switch  Criteria=u2 > Threshold  SaturateOnIntegerOverflow=off  InputSameDT=off
  AccelerationToDeceleration : Gain  Gain=-1  ParamDataTypeStr=double
  AccelerationToDownHill : Sum  Inputs=+-
  AccelerationToUpHill : Sum  Inputs=+-
  DecelerationSwitch : Switch  Criteria=u2 > Threshold  SaturateOnIntegerOverflow=off  InputSameDT=off
  DecelerationToDownHill : Sum
  DecelerationToUpHill : Sum
  DivisionByVelocity : Product
  ForceToAcceleration : Product  Inputs=*/  OutDataTypeStr=double
  GreaterThan : RelationalOperator  Operator=>  OutDataTypeStr=boolean  RndMeth=Simplest  InputSameDT=off
  LimitMaxAcceleration : MATLAB Function  TreatAsAtomicUnit=on
  RoadResistForceSubtraction : Sum  Inputs=+-
  SelectMin : Switch  Criteria=u2 > Threshold  OutDataTypeStr=double  SaturateOnIntegerOverflow=off  InputSameDT=off
  SelectVelocityOrNot : Switch  Criteria=u2 > Threshold  OutDataTypeStr=double  SaturateOnIntegerOverflow=off  InputSameDT=off
  TractionPower : Product  OutDataTypeStr=double
  ZeroReplacedByDecimal : MATLAB Function  TreatAsAtomicUnit=on
  AccelerationOut : Outport  OutDataTypeStr=double  OutputWhenDisabled=reset  InitialOutput=0
  DecelerationOut : Outport  Port=2  OutDataTypeStr=double  OutputWhenDisabled=reset  InitialOutput=0
  wires:
  PowerRelative/1 -> TractionPower/2
  PowerMaximum/1 -> TractionPower/1
  TractionPower/1 -> SelectMin/3, GreaterThan/1
  TractionForce/1 -> SelectMin/1, GreaterThan/2
  SelectMin/1 -> RoadResistForceSubtraction/1
  Gradient/1 -> AccelerationSwitch/2, DecelerationSwitch/2, AccelerationGravity/1
  GravitationalAcceleration/1 -> AccelerationGravity/2
  ForceToAcceleration/1 -> DecelerationToDownHill/1, AccelerationToDownHill/1, DecelerationToUpHill/1, AccelerationToUpHill/1
  AccelerationGravity/1 -> DecelerationToUpHill/2, AccelerationToUpHill/2, DecelerationToDownHill/2, AccelerationToDownHill/2
  RoadResistForceSubtraction/1 -> ForceToAcceleration/1
  DecelerationToUpHill/1 -> DecelerationSwitch/1
  AccelerationToUpHill/1 -> AccelerationSwitch/1
  AccelerationToDeceleration/1 -> DecelerationOut/1
  AccelerationToDownHill/1 -> AccelerationSwitch/3
  DecelerationToDownHill/1 -> DecelerationSwitch/3
  RoadResistTotalIn/1 -> RoadResistForceSubtraction/2
  VelocityFinalFeedback/1 -> ZeroReplacedByDecimal/1(u)
  ZeroReplacedByDecimal/1(y) -> DivisionByVelocity/1
  GreaterThan/1 -> SelectVelocityOrNot/2, SelectMin/2
  DivisionByVelocity/1 -> SelectVelocityOrNot/3
  WeightOfTrainIn/1 -> SelectVelocityOrNot/1, DivisionByVelocity/2
  SelectVelocityOrNot/1 -> ForceToAcceleration/2
  DecelerationSwitch/1 -> LimitMaxAcceleration/2(u2)
  LimitMaxAcceleration/2(y2) -> AccelerationToDeceleration/1
  LimitMaxAcceleration/1(y1) -> AccelerationOut/1
  AccelerationSwitch/1 -> LimitMaxAcceleration/1(u1)

== system simulator/TrainSimulator/AccToForceAndForceToAcc/VehicleResist ==
  VehicleResisIn : Inport  OutMin=0  OutDataTypeStr=double
  VehicleResisOut : Outport  OutMin=0  OutDataTypeStr=double
  wires:
  VehicleResisIn/1 -> VehicleResisOut/1

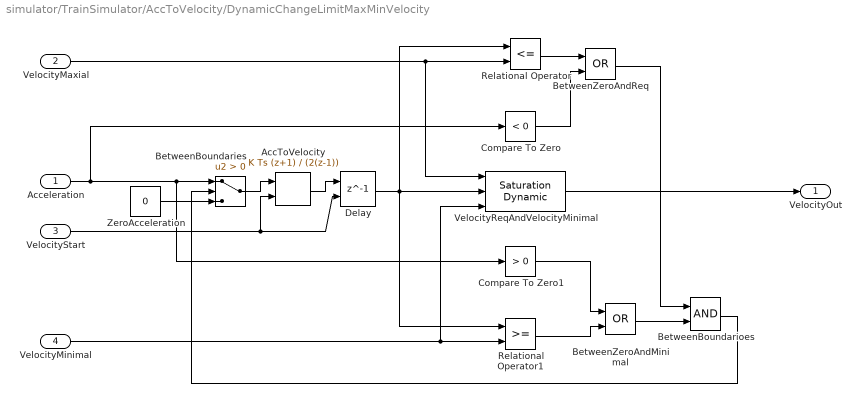
== system simulator/TrainSimulator/AccToVelocity/DynamicChangeLimitMaxMinVelocity ==
  Acceleration : Inport  OutDataTypeStr=double
  VelocityMaxial : Inport  Port=2  OutDataTypeStr=double
  VelocityStart : Inport  Port=3  OutDataTypeStr=double
  VelocityMinimal : Inport  Port=4  OutDataTypeStr=double
  AccToVelocity : DiscreteIntegrator  IntegratorMethod=Integration: Trapezoidal  InitialConditionSource=external  SampleTime=-1  OutDataTypeStr=double  UpperSaturationLimit=50  LowerSaturationLimit=0  ICPrevOutput=DiscIntNeverNeededParam  ICPrevScaledInput=DiscIntNeverNeededParam
  BetweenBoundaries : Switch  Criteria=u2 > Threshold  OutDataTypeStr=double  SaturateOnIntegerOverflow=off  InputSameDT=off
  BetweenBoundarioes : Logic  AllPortsSameDT=off  OutDataTypeStr=boolean
  BetweenZeroAndMinimal : Logic  Operator=OR  AllPortsSameDT=off  OutDataTypeStr=boolean
  BetweenZeroAndReq : Logic  Operator=OR  AllPortsSameDT=off  OutDataTypeStr=boolean
  Compare To Zero : simulink/Logic and Bit Operations/Compare To Zero  relop=<  OutDataTypeStr=boolean  ZeroCross=off
  Compare To Zero1 : simulink/Logic and Bit Operations/Compare To Zero  relop=>  OutDataTypeStr=boolean  ZeroCross=off
  Delay : Delay  DelayLength=1  InitialConditionSource=Input port
      settings: InputPortMap=u0,p4
  Relational Operator : RelationalOperator  Operator=<=  OutDataTypeStr=boolean  InputSameDT=off
  Relational Operator1 : RelationalOperator  OutDataTypeStr=boolean  InputSameDT=off
  VelocityReqAndVelocityMinimal : simulink/Discontinuities/Saturation Dynamic  OutMin=[]  OutMax=[]  OutDataTypeStr=double  OutDataType=fixdt(1, 16)  OutScaling=2^-10  RndMeth=Nearest  DoSatur=off
  ZeroAcceleration : Constant  Value=0  OutDataTypeStr=uint8
  VelocityOut : Outport  OutDataTypeStr=double
  wires:
  Acceleration/1 -> Compare To Zero1/1, BetweenBoundaries/1, Compare To Zero/1
  ZeroAcceleration/1 -> BetweenBoundaries/3
  BetweenBoundaries/1 -> AccToVelocity/1
  Relational Operator/1 -> BetweenZeroAndReq/1
  Compare To Zero/1 -> BetweenZeroAndReq/2
  VelocityMaxial/1 -> Relational Operator/2, VelocityReqAndVelocityMinimal/1
  VelocityMinimal/1 -> Relational Operator1/2, VelocityReqAndVelocityMinimal/3
  Compare To Zero1/1 -> BetweenZeroAndMinimal/1
  Relational Operator1/1 -> BetweenZeroAndMinimal/2
  BetweenZeroAndMinimal/1 -> BetweenBoundarioes/2
  BetweenZeroAndReq/1 -> BetweenBoundarioes/1
  BetweenBoundarioes/1 -> BetweenBoundaries/2
  VelocityReqAndVelocityMinimal/1 -> VelocityOut/1
  Delay/1 -> Relational Operator1/1, Relational Operator/1, VelocityReqAndVelocityMinimal/2
  VelocityStart/1 -> Delay/2, AccToVelocity/2
  AccToVelocity/1 -> Delay/1

== system simulator/TrainSimulator/AccelerationCalculating/BreakCurves ==
  AccelerationIn : Inport  OutDataTypeStr=double
  Action Port : ActionPort  ActionPortLabel=case [ 4 ]:
  AccelerationOut : Outport  OutDataTypeStr=double  InitialOutput=0
  wires:
  AccelerationIn/1 -> AccelerationOut/1

== system simulator/TrainSimulator/AccelerationCalculating/ConstantAcceleration ==
  AccelerationIn : Inport  OutDataTypeStr=double
  Action Port : ActionPort  ActionPortLabel=case [ 3 ]:
  AccelerationOut : Outport  OutDataTypeStr=double  InitialOutput=0
  wires:
  AccelerationIn/1 -> AccelerationOut/1

== system simulator/TrainSimulator/AccelerationCalculating/ConstantVelocity ==
  Action Port : ActionPort  ActionPortLabel=case [ 1 ]:
  ZeroAcceleration : Constant  Value=0  OutMin=0  OutMax=0  OutDataTypeStr=double
  AccelerationOut : Outport  OutDataTypeStr=double  InitialOutput=0
  wires:
  ZeroAcceleration/1 -> AccelerationOut/1

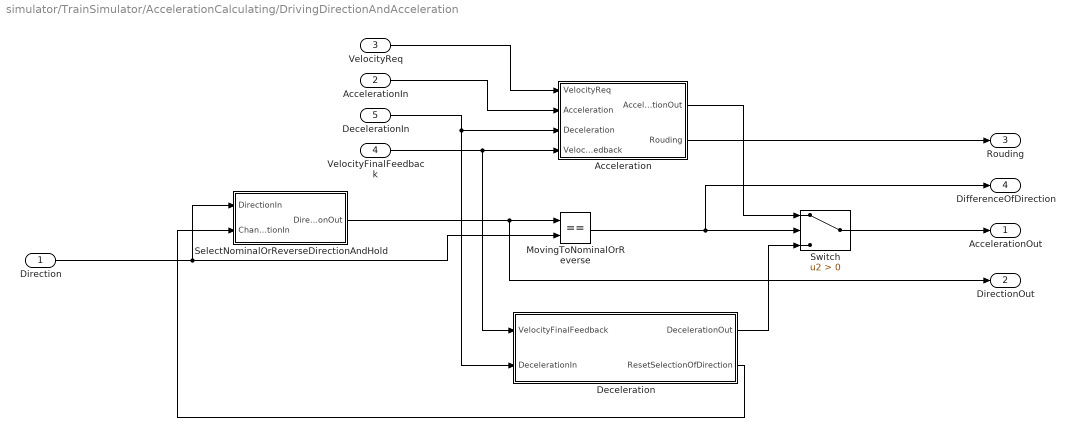
== system simulator/TrainSimulator/AccelerationCalculating/DrivingDirectionAndAcceleration ==
  Direction : Inport  OutDataTypeStr=uint8
  AccelerationIn : Inport  Port=2  OutDataTypeStr=double
  VelocityReq : Inport  Port=3  OutDataTypeStr=double
  VelocityFinalFeedback : Inport  Port=4  OutDataTypeStr=double
  DecelerationIn : Inport  Port=5  OutDataTypeStr=double
  Acceleration : Subsystem
  Deceleration : Subsystem
  MovingToNominalOrReverse : RelationalOperator  Operator===  OutDataTypeStr=boolean  RndMeth=Simplest  InputSameDT=off
  SelectNominalOrReverseDirectionAndHold : Subsystem
  Switch : Switch  Criteria=u2 > Threshold  OutDataTypeStr=double  SaturateOnIntegerOverflow=off  InputSameDT=off
  AccelerationOut : Outport  OutDataTypeStr=double  OutputWhenDisabled=reset  InitialOutput=0
  DirectionOut : Outport  Port=2  OutDataTypeStr=uint8  OutputWhenDisabled=reset  InitialOutput=0
  Rouding : Outport  Port=3  OutDataTypeStr=double
  DifferenceOfDirection : Outport  Port=4  OutDataTypeStr=boolean
  wires:
  Direction/1 -> MovingToNominalOrReverse/2, SelectNominalOrReverseDirectionAndHold/1(DirectionIn)
  SelectNominalOrReverseDirectionAndHold/1(DirectionOut) -> DirectionOut/1, MovingToNominalOrReverse/1
  MovingToNominalOrReverse/1 -> DifferenceOfDirection/1, Switch/2
  Deceleration/1(DecelerationOut) -> Switch/3
  Acceleration/1(AccelerationOut) -> Switch/1
  Switch/1 -> AccelerationOut/1
  VelocityFinalFeedback/1 -> Deceleration/1(VelocityFinalFeedback), Acceleration/4(VelocityFinalFeedback)
  VelocityReq/1 -> Acceleration/1(VelocityReq)
  Deceleration/2(ResetSelectionOfDirection) -> SelectNominalOrReverseDirectionAndHold/2(ChangeDirectionIn)
  DecelerationIn/1 -> Acceleration/3(Deceleration), Deceleration/2(DecelerationIn)
  AccelerationIn/1 -> Acceleration/2(Acceleration)
  Acceleration/2(Rouding) -> Rouding/1

== system simulator/TrainSimulator/AccelerationCalculating/SuddenChangeOfVelocity ==
  VelocityReq : Inport  OutDataTypeStr=double
  VelocityFinalFeedback : Inport  Port=2  OutDataTypeStr=double
  Action Port : ActionPort  ActionPortLabel=case [ 2 ]:
  Relational Operator1 : RelationalOperator  Operator=>  OutDataTypeStr=boolean  RndMeth=Simplest  InputSameDT=off
  Relational Operator2 : RelationalOperator  Operator=<  OutDataTypeStr=boolean  RndMeth=Simplest  InputSameDT=off
  SuddenChangeofSpeedToMax : Constant  Value=100000  OutDataTypeStr=uint32
  SuddenChangeofSpeedToMin : Constant  Value=100000  OutDataTypeStr=uint32
  Sum : Sum  Inputs=|++  OutDataTypeStr=double  AccumDataTypeStr=double
  Switch : Switch  Criteria=u2 > Threshold  OutDataTypeStr=double  SaturateOnIntegerOverflow=off  InputSameDT=off
  Switch1 : Switch  Criteria=u2 > Threshold  OutDataTypeStr=double  SaturateOnIntegerOverflow=off  InputSameDT=off
  ZeroAccelerationToMax : Constant  Value=0  OutDataTypeStr=uint8
  ZeroAccelerationToMin : Constant  Value=0  OutDataTypeStr=uint8
  AccelerationOut : Outport  OutDataTypeStr=double  InitialOutput=0
  wires:
  VelocityFinalFeedback/1 -> Relational Operator2/2, Relational Operator1/2
  SuddenChangeofSpeedToMax/1 -> Switch/1
  Relational Operator1/1 -> Switch/2
  VelocityReq/1 -> Relational Operator2/1, Relational Operator1/1
  ZeroAccelerationToMax/1 -> Switch/3
  Relational Operator2/1 -> Switch1/2
  SuddenChangeofSpeedToMin/1 -> Switch1/1
  ZeroAccelerationToMin/1 -> Switch1/3
  Sum/1 -> AccelerationOut/1
  Switch/1 -> Sum/1
  Switch1/1 -> Sum/2

== system simulator/TrainSimulator/AccelerationCalculating/TractionCharacteristics ==
  AccelerationIn : Inport  OutDataTypeStr=double
  Action Port : ActionPort  ActionPortLabel=case [ 5 ]:
  AccelerationOut : Outport  OutDataTypeStr=double  InitialOutput=0
  wires:
  AccelerationIn/1 -> AccelerationOut/1
